simulink library "speedgoatlib_IO682_3210"  (R2024b)
settings: Solver=FixedStepAuto  StartTime=0.0  StopTime=10.0  RelTol=1e-3  EnableMultiTasking=on
undefined symbols (not defined in the file): sg_io682_receive_decode_m_v2
libraries: speedgoatlib_obsolete x1
settings Model: Creator=cschafft  LastModifiedBy=speedgoat\jenkins
settings SolverCC: ConcurrentTasks=on  AlgebraicLoopSolver=TrustRegion  AutoInsertRateTranBlk=on  InsertRTBMode=Never (minimum delay)
settings DataIOCC: LimitDataPoints=on  SaveFormat=StructureWithTime  ReturnWorkspaceOutputs=off
settings OptimizationCC: BlockReduction=off  OptimizeBlockIOStorage=off  BufferReuse=off  ReuseModelBlockBuffer=off  GlobalBufferReuse=off  ExpressionFolding=off  LocalBlockOutputs=off  OptimizeDataStoreBuffers=off  BusAssignmentInplaceUpdate=off
settings DebuggingCC: UnconnectedInputMsg=warning  UnconnectedOutputMsg=warning  UnconnectedLineMsg=warning  AllowSymbolicDim=off  SFUnexpectedBacktrackingDiag=warning  SFNoUnconditionalDefaultTransitionDiag=warning  SFExecutionAtInitializationDiag=none  ArithmeticOperatorsInVariantConditions=warning
settings HardwareCC: ProdBitPerPointer=32  ProdBitPerSizeT=32  ProdBitPerPtrDiffT=32  ProdLargestAtomicFloat=None  ProdWordSize=32  ProdLongLongMode=on  ProdHWDeviceType=Generic->32-bit x86 compatible
settings ModelReferenceCC: EnableRefExpFcnMdlSchedulingChecks=on  PropagateSignalLabelsOutOfModel=off
settings SFSimCC: SimUseLocalCustomCode=off  CustomCodeUndefinedFunction=UseInterfaceOnly
settings RTWCC: Description=Simulink Real-Time  SystemTargetFile=slrt.tlc  TemplateMakefile=slrt_default_tmf  RTWUseLocalCustomCode=off  RTWCompilerOptimization=on  GPUComputeCapability=3.5  DLArmComputeVersion=19.05
settings CodeAppCC: StateflowObjectComments=on
settings SimulinkRealTimeCC: SubcomponentCodeInterfacePackaging=Reusable function  SupportVariableSizeSignals=on  InstructionSetFMA=off  OptimizeReductions=off  LogToMDFFile=off  RL32LogTETModifier=off
settings ConfigComp: CovMetricSettings=dw  CovSaveCumulativeToWorkspaceVar=on  CovSaveSingleToWorkspaceVar=on  CovExternalEMLEnable=off  CovBoundaryAbsTol=1.0e-5

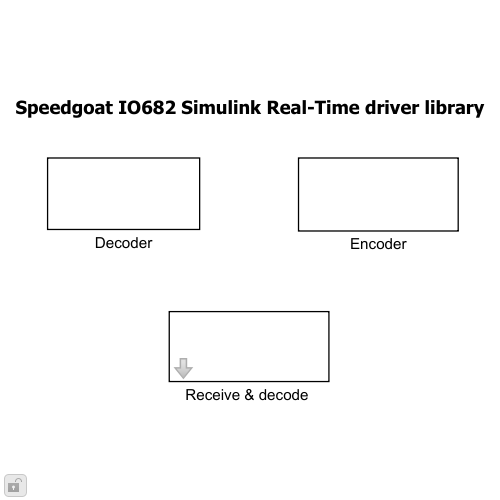
[thumbnail: Simulink's stored preview of the top-level diagram]
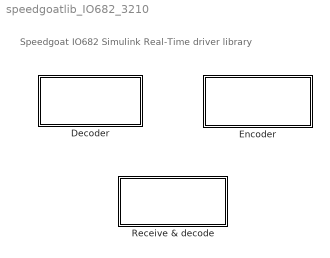
== system speedgoatlib_IO682_3210 ==
  note: Speedgoat IO682 Simulink Real-Time driver library
  Decoder : Subsystem
  Encoder : Subsystem
  "Receive & decode " : Subsystem  InitFcn=sg_io682_receive_decode_m_v2.runInitFcn();  mask(receive_decode_IO682){parChannel=1, parImportedIcdFile=, parSampleTime=-1, parSelectedLabels=[]}
      mask prompts: parChannel "Channel"; parImportedIcdFile "Available Messages (*.csv)"; parSampleTime "Sample Time [s]"
      mask help:
      | Receive and decode data from ARINC 429.
      | Use the "Select Messages to Decode" button to select the messages to decode, the block will automatically configure itself based on label name. The message description is given by the ICD file defined in "Available Messages".
      mask init:
      | sg_io682_receive_decode_m_v2.runMaskInitialization();
      settings: CopyFcn=sg_io682_receive_decode_m_v2.runCopyFcn();
      mask TypeOptions parChannel: Receive v2 /parChannel
      mask TypeOptions parSampleTime: Receive v2 /parSampleTime
      mask DialogControl parImportIcdFile Prompt: Browse
      mask DialogControl parImportIcdFile Callback: sg_io682_receive_decode_m_v2.runImportIcdFileCb();
      mask DialogControl parSelectLabels Prompt: Select Messages to Decode
      mask DialogControl parSelectLabels Callback: sg_io682_receive_decode_m_v2.runSelectLabelsCb();

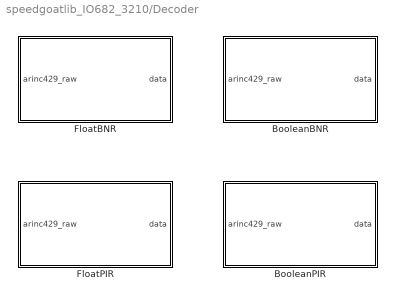
== system speedgoatlib_IO682_3210/Decoder ==
  BooleanBNR : Subsystem  mask(Boolean BNR Decoder){label=0, float_resolution=0, signal_lsb=0, signal_msb=0}
      mask prompts: float_resolution "Float Resolution"; signal_lsb "Signal LSB"; signal_msb "Signal MSB"
      mask help: Decode an ARINC message in BNR format of boolean data type.
  BooleanPIR : Subsystem  mask(Boolean PIR Decoder){label=0, float_resolution=0, signal_lsb=0, signal_msb=0}
      mask prompts: float_resolution "Float Resolution"; signal_lsb "Signal LSB"; signal_msb "Signal MSB"
      mask help: Decode an ARINC message of boolean data type when encoded as "Parameter In Demand" (PIR) using IEEE encoding.
  FloatBNR : Subsystem  mask(Float BNR Decoder){label=0, float_resolution=0, signal_lsb=0, signal_msb=0}
      mask prompts: float_resolution "Float Resolution"; signal_lsb "Signal LSB"; signal_msb "Signal MSB"
      mask help: Decode an ARINC message in BNR format of float data type.
  FloatPIR : Subsystem  mask(Float PIR Decoder){label=0, float_resolution=0, signal_lsb=0, signal_msb=0}
      mask prompts: float_resolution "Float Resolution"; signal_lsb "Signal LSB"; signal_msb "Signal MSB"
      mask help: Decode an ARINC message of float data type when encoded as "Parameter In Demand" (PIR) using IEEE encoding.

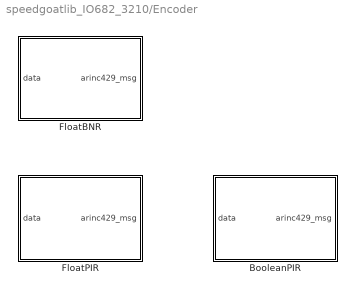
== system speedgoatlib_IO682_3210/Encoder ==
  BooleanPIR : Subsystem  mask(Boolean PIR Encoder){label=0, SSM=0, SDI=0}
      mask help: Encode an ARINC message from a boolean data as a "Parameter In Demand" (PIR) using the IEEE encoding.
  FloatBNR : Subsystem  mask(Float BNR Encoder){label=0, SSM=0, SDI=0, float_resolution=0, signal_lsb=0, signal_msb=0}
      mask prompts: float_resolution "Float Resolution"; signal_lsb "Signal LSB"; signal_msb "Signal MSB"
      mask help: Encode an ARINC message from a float data using the BNR encoding.
  FloatPIR : Subsystem  mask(Float PIR Encoder){label=0}
      mask help: Encode an ARINC message from a float data as a "Parameter In Demand" (PIR) using the IEEE encoding.

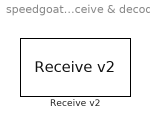
== system speedgoatlib_IO682_3210/Receive & decode  ==
  "Receive v2 " : speedgoatlib_obsolete/IO682/Receive v2   parModuleId=1  parChannel=1  parMaxWords=50  parMinWords=1  parSampleTime=parSampleTime

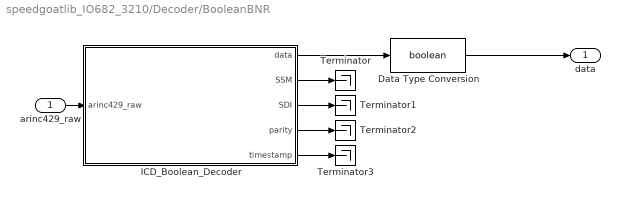
== system speedgoatlib_IO682_3210/Decoder/BooleanBNR ==
  arinc429_raw : Inport
  Data Type Conversion : DataTypeConversion  OutDataTypeStr=boolean  SaturateOnIntegerOverflow=off  RndMeth=Floor
  ICD_Boolean_Decoder : MATLAB Function  TreatAsAtomicUnit=on  VariantControl=mode==99
  Terminator{,1..3} (4 alike) : Terminator
  data : Outport  VectorParamsAs1DForOutWhenUnconnected=off
  wires:
  arinc429_raw/1 -> ICD_Boolean_Decoder/1(arinc429_raw)
  ICD_Boolean_Decoder/1(data) -> Data Type Conversion/1
  ICD_Boolean_Decoder/2(SSM) -> Terminator/1
  ICD_Boolean_Decoder/3(SDI) -> Terminator1/1
  ICD_Boolean_Decoder/4(parity) -> Terminator2/1
  ICD_Boolean_Decoder/5(timestamp) -> Terminator3/1
  Data Type Conversion/1 -> data/1

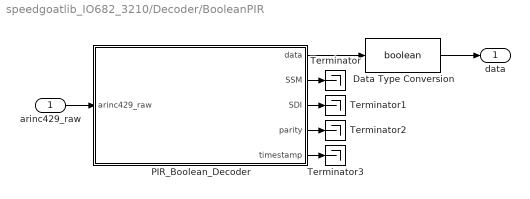
== system speedgoatlib_IO682_3210/Decoder/BooleanPIR ==
  arinc429_raw : Inport
  Data Type Conversion : DataTypeConversion  OutDataTypeStr=boolean  SaturateOnIntegerOverflow=off  RndMeth=Floor
  PIR_Boolean_Decoder : MATLAB Function  TreatAsAtomicUnit=on
  Terminator{,1..3} (4 alike) : Terminator
  data : Outport  VectorParamsAs1DForOutWhenUnconnected=off
  wires:
  arinc429_raw/1 -> PIR_Boolean_Decoder/1(arinc429_raw)
  PIR_Boolean_Decoder/2(SSM) -> Terminator/1
  PIR_Boolean_Decoder/1(data) -> Data Type Conversion/1
  PIR_Boolean_Decoder/3(SDI) -> Terminator1/1
  PIR_Boolean_Decoder/4(parity) -> Terminator2/1
  PIR_Boolean_Decoder/5(timestamp) -> Terminator3/1
  Data Type Conversion/1 -> data/1

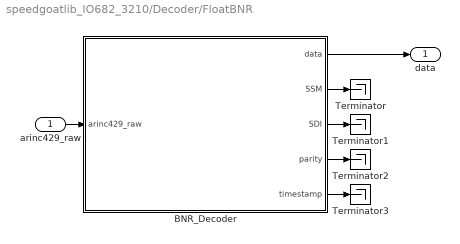
== system speedgoatlib_IO682_3210/Decoder/FloatBNR ==
  arinc429_raw : Inport
  BNR_Decoder : MATLAB Function  TreatAsAtomicUnit=on  VariantControl=mode==99
  Terminator{,1..3} (4 alike) : Terminator
  data : Outport  VectorParamsAs1DForOutWhenUnconnected=off
  wires:
  BNR_Decoder/5(timestamp) -> Terminator3/1
  BNR_Decoder/1(data) -> data/1
  BNR_Decoder/2(SSM) -> Terminator/1
  BNR_Decoder/3(SDI) -> Terminator1/1
  arinc429_raw/1 -> BNR_Decoder/1(arinc429_raw)
  BNR_Decoder/4(parity) -> Terminator2/1

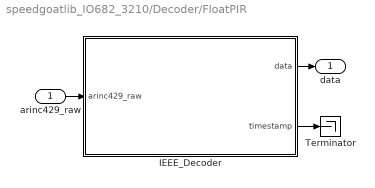
== system speedgoatlib_IO682_3210/Decoder/FloatPIR ==
  arinc429_raw : Inport
  IEEE_Decoder : MATLAB Function  TreatAsAtomicUnit=on
  Terminator : Terminator
  data : Outport  VectorParamsAs1DForOutWhenUnconnected=off
  wires:
  IEEE_Decoder/1(data) -> data/1
  arinc429_raw/1 -> IEEE_Decoder/1(arinc429_raw)
  IEEE_Decoder/2(timestamp) -> Terminator/1

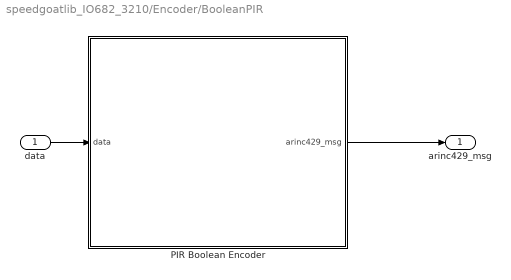
== system speedgoatlib_IO682_3210/Encoder/BooleanPIR ==
  data : Inport
  PIR Boolean Encoder : MATLAB Function  TreatAsAtomicUnit=on
  arinc429_msg : Outport  VectorParamsAs1DForOutWhenUnconnected=off
  wires:
  PIR Boolean Encoder/1(arinc429_msg) -> arinc429_msg/1
  data/1 -> PIR Boolean Encoder/1(data)

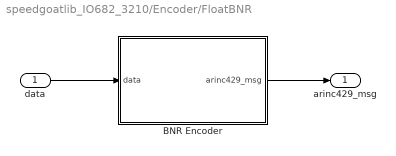
== system speedgoatlib_IO682_3210/Encoder/FloatBNR ==
  data : Inport
  BNR Encoder : MATLAB Function  TreatAsAtomicUnit=on
  arinc429_msg : Outport  VectorParamsAs1DForOutWhenUnconnected=off
  wires:
  data/1 -> BNR Encoder/1(data)
  BNR Encoder/1(arinc429_msg) -> arinc429_msg/1

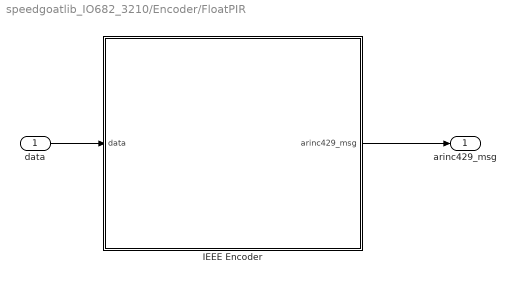
== system speedgoatlib_IO682_3210/Encoder/FloatPIR ==
  data : Inport
  IEEE Encoder : MATLAB Function  TreatAsAtomicUnit=on
  arinc429_msg : Outport  VectorParamsAs1DForOutWhenUnconnected=off
  wires:
  data/1 -> IEEE Encoder/1(data)
  IEEE Encoder/1(arinc429_msg) -> arinc429_msg/1

== matlab function speedgoatlib_IO682_3210/Decoder/FloatBNR/BNR_Decoder ==
  data: arinc429_raw input double; label parameter int32; data output size=[1, 1]; float_resolution parameter double size=[1, 1]; signal_lsb parameter int32 size=[1, 1]; signal_msb parameter int32 size=[1, 1]; SSM output; SDI output; parity output; timestamp output
% Function description: this function takes a vector of ARINC429 as inputs
% and decodes its content.
%
% 
%
%
function [data,SSM,SDI,parity,timestamp] = fcn(arinc429_raw, label, float_resolution, signal_lsb, signal_msb)
%#codegen

persistent data_buf;
persistent SDI_buf;
persistent SSM_buf;
persistent timestamp_buf;

if isempty(data_buf)
    data_buf = double(0.0);
end

if isempty(SDI_buf)
    SDI_buf = double(0.0);
end

if isempty(SSM_buf)
    SSM_buf = double(0.0);
end

if isempty(timestamp_buf)
    timestamp_buf = double(0.0);
end
    

% We process all the inputs messages and if the labels matches, then the
% buffered variables (_buf) are updated.

% When no label match, we keep the values of the previous execution
for i = 1:length(arinc429_raw)

    arinc429_raw_64 = typecast(arinc429_raw(i), 'uint64');
    arinc429_raw_32_low = uint32(bitand(arinc429_raw_64, 2^32-1));
    arinc429_raw_32_high = uint32(bitand(bitshift(arinc429_raw_64, -32), 2^32-1));

    label_field = int32(bitand(arinc429_raw_32_low, uint32(255)));

    if label_field == label

        % Index the bits position from offset 0.
        signal_lsb = signal_lsb - 1;
        signal_msb = signal_msb - 1;
        signal_range = signal_msb - signal_lsb + 1;

        % Get the sign (bit 29)
        sign = bitand(bitshift(arinc429_raw_32_low, -signal_msb -1), 1);

        % Get the data field
        data_bnr_mask = uint32(2^(signal_range) - 1);
        data_bnr = uint32(arinc429_raw_32_low);
        data_bnr = bitand(bitshift(data_bnr, -signal_lsb), data_bnr_mask);        

        % If needed, pad the sign bit (we work on 32-bits)
        if sign > 0
            % fill all the bits between sign and MSB with logic 1
            padding_bits = uint32(bitshift(uint32(2^(32 - signal_range) - 1), signal_range));
            data_bnr_signed = typecast(bitor(data_bnr, padding_bits), 'int32');
        else
            data_bnr_signed = typecast(data_bnr, 'int32');    
        end
        
        % Get the SSM field
        SSM_buf = double(bitand(bitshift(arinc429_raw_32_low, -29), 3));
        
        % Get the SDI field
        SDI_buf = double(bitand(bitshift(arinc429_raw_32_low, -8), 3));

        % Update the data only when labels match
        data_buf = double(float_resolution * double(data_bnr_signed));
        timestamp_buf = double(arinc429_raw_32_high);


    end

end


% Update the output using the buffered values.
data = data_buf;
SSM = SSM_buf;
SDI = SDI_buf;
parity = -1.0;
timestamp = timestamp_buf;

== matlab function speedgoatlib_IO682_3210/Decoder/FloatPIR/IEEE_Decoder ==
  data: data output double size=[1, 1]; arinc429_raw input double; timestamp output; label parameter
function [data, timestamp]  = fcn(arinc429_raw, label)
%#codegen

% Function description: this function takes a vector of ARINC429 as inputs
% and decodes its content.

persistent data_buf;
persistent timestamp_buf;

if isempty(data_buf)
    data_buf = double(0.0);
end
    

if isempty(timestamp_buf)
    timestamp_buf = double(0.0);
end
    

% We process all the inputs messages and if the labels matches, then the
% buffered variables (_buf) are updated.

% When no label match, we keep the values of the previous execution
for i = 1:length(arinc429_raw)

    arinc429_raw_64 = typecast(arinc429_raw(i), 'uint64');
    arinc429_raw_32_low = uint32(bitand(arinc429_raw_64, 2^32-1));
    arinc429_raw_32_high = uint32(bitand(bitshift(arinc429_raw_64, -32), 2^32-1));

    label_field = int32(bitand(arinc429_raw_32_low, uint32(255)));

    if label_field == label

        % Get the sign (bit 31)
        sign = bitand(bitshift(arinc429_raw_32_low, -30), 1);

        % Get the exponent and the mantissa
        exponent =  int32(bitand(bitshift(arinc429_raw_32_low, -22), 255)) - 127;        
        mantissa_bnr = uint32(bitand(bitshift(arinc429_raw_32_low, -8), 2^14-1));
        mantissa = 0.0;
        for j = 1:14
            if bitand(mantissa_bnr, 8192)
                mantissa = mantissa + 2^(-j);
            end
            mantissa_bnr = bitshift(mantissa_bnr, 1);
        end
        mantissa = mantissa + 1;
        
        % Update the data only when labels match
        data_buf = double((-1.0)^double(sign) * 2^(double(exponent)) * double(mantissa));
        timestamp_buf = double(arinc429_raw_32_high);


    end

end


% Update the output using the buffered values.
data = data_buf;
timestamp = timestamp_buf;

== matlab function speedgoatlib_IO682_3210/Decoder/BooleanBNR/ICD_Boolean_Decoder ==
  data: arinc429_raw input double; label parameter int32; data output size=[1, 1]; signal_lsb parameter int32 size=[1, 1]; signal_msb parameter int32 size=[1, 1]; SSM output; SDI output; parity output; timestamp output
% Function description: this function takes a vector of ARINC429 as inputs
% and decodes its content.
%
% 
%
%
function [data,SSM,SDI,parity,timestamp] = fcn(arinc429_raw, label, signal_lsb, signal_msb)
%#codegen

persistent data_buf;
persistent SDI_buf;
persistent SSM_buf;
persistent timestamp_buf;

if isempty(data_buf)
    data_buf = double(0.0);
end

if isempty(SDI_buf)
    SDI_buf = double(0.0);
end

if isempty(SSM_buf)
    SSM_buf = double(0.0);
end

if isempty(timestamp_buf)
    timestamp_buf = double(0.0);
end
    

% We process all the inputs messages and if the labels matches, then the
% buffered variables (_buf) are updated.

% When no label match, we keep the values of the previous execution
for i = 1:length(arinc429_raw)

    arinc429_raw_64 = typecast(arinc429_raw(i), 'uint64');
    arinc429_raw_32_low = uint32(bitand(arinc429_raw_64, 2^32-1));
    arinc429_raw_32_high = uint32(bitand(bitshift(arinc429_raw_64, -32), 2^32-1));

    label_field = int32(bitand(arinc429_raw_32_low, uint32(255)));

    if label_field == label

        % Index the bits position from offset 0.
        signal_lsb = signal_lsb - 1;
        signal_msb = signal_msb - 1;
        signal_range = signal_msb - signal_lsb + 1;

        % Get the sign (bit 29)
        sign = bitand(bitshift(arinc429_raw_32_low, -signal_msb -1), 1);

        % Get the data field
        data_bnr_mask = uint32(2^(signal_range) - 1);
        data_bnr = uint32(arinc429_raw_32_low);
        data_bnr = bitand(bitshift(data_bnr, -signal_lsb), data_bnr_mask);        

        % If needed, pad the sign bit (we work on 32-bits)
        if sign > 0
            % fill all the bits between sign and MSB with logic 1
            padding_bits = uint32(bitshift(uint32(2^(32 - signal_range) - 1), signal_range));
            data_bnr_signed = typecast(bitor(data_bnr, padding_bits), 'int32');
        else
            data_bnr_signed = typecast(data_bnr, 'int32');    
        end
        
        % Get the SSM field
        SSM_buf = double(bitand(bitshift(arinc429_raw_32_low, -29), 3));
        
        % Get the SDI field
        SDI_buf = double(bitand(bitshift(arinc429_raw_32_low, -8), 3));

        % Update the data only when labels match       
        data_buf = double(double(data_bnr_signed));
        timestamp_buf = double(arinc429_raw_32_high);


    end

end

% Update the output using the buffered values.
data = data_buf;
SSM = SSM_buf;
SDI = SDI_buf;
parity = -1.0;
timestamp = timestamp_buf;

== matlab function speedgoatlib_IO682_3210/Encoder/BooleanPIR/PIR Boolean Encoder ==
  data: data input double size=[1, 1]; arinc429_msg output double size=[1, 1]; SSM parameter uint32 size=[1, 1]; SDI parameter uint32 size=[1, 1]; label parameter uint32 size=[1, 1]
function arinc429_msg = fcn(data, SSM, SDI, label)
%#codegen
% Scale the data using the float resolution parameter.

if data > 0.5
    data_32 = uint32(2^21);
else
    data_32 = uint32(0);
end   

label = bitand(label, bin2dec('00000000000000000000000011111111'));
SDI = bitand(SDI, bin2dec('00000000000000000000000000000011'));
SSM = bitand(SSM, bin2dec('00000000000000000000000000000011'));

arinc429_32 = uint32(bitor(bitshift(SSM, 29), bitor(bitshift(SDI, 8), bitor(data_32, label))));
arinc429_64 = uint64(arinc429_32);
arinc429_msg = typecast(arinc429_64, 'double');

== matlab function speedgoatlib_IO682_3210/Encoder/FloatBNR/BNR Encoder ==
  data: data input double size=[1, 1]; arinc429_msg output double size=[1, 1]; SSM parameter uint32 size=[1, 1]; SDI parameter uint32 size=[1, 1]; label parameter uint32 size=[1, 1]; float_resolution parameter; signal_lsb parameter; signal_msb parameter
function arinc429_msg = bnr_encoder(data, SSM, SDI, label, float_resolution, signal_lsb, signal_msb)
%#codegen
% Scale the data using the float resolution parameter.
signal_lsb = signal_lsb - 1;
data_32 = typecast(int32(data / float_resolution), 'uint32');
data_32 = bitshift(data_32, signal_lsb);    

label = bitand(label, bin2dec('00000000000000000000000011111111'));
SDI = bitand(SDI, bin2dec('00000000000000000000000000000011'));
SSM = bitand(SSM, bin2dec('00000000000000000000000000000011'));

arinc429_32 = uint32(bitor(bitshift(SSM, 29), bitor(bitshift(SDI, 8), bitor(data_32, label))));
sign = bitand(bitshift(arinc429_32, -28), 1)
arinc429_64 = uint64(arinc429_32);
arinc429_msg = typecast(arinc429_64, 'double');

== matlab function speedgoatlib_IO682_3210/Decoder/BooleanPIR/PIR_Boolean_Decoder ==
  data: arinc429_raw input double; label parameter uint32; data output size=[1, 1]; SSM output double size=[1, 1]; SDI output double size=[1, 1]; parity output double size=[1, 1]; timestamp output
% Function description: this function takes a vector of ARINC429 as inputs
% and decodes its content.
%
% 
%
%
function [data, SSM, SDI, parity, timestamp] = fcn(arinc429_raw, label)
%#codegen
bool_pos = 22 - 1;
persistent data_buf;
persistent SDI_buf;
persistent SSM_buf;
persistent timestamp_buf;

if isempty(data_buf)
    data_buf = false;
end

if isempty(SDI_buf)
    SDI_buf = double(0.0);
end

if isempty(SSM_buf)
    SSM_buf = double(0.0);
end

if isempty(timestamp_buf)
    timestamp_buf = double(0.0);
end
    

% We process all the inputs messages and if the labels matches, then the
% buffered variables (_buf) are updated.

% When no label match, we keep the values of the previous execution
for i = 1:length(arinc429_raw)

    arinc429_raw_64 = typecast(arinc429_raw(i), 'uint64');
    arinc429_raw_32_low = uint32(bitand(arinc429_raw_64, 2^32-1));
    arinc429_raw_32_high = uint32(bitand(bitshift(arinc429_raw_64, -32), 2^32-1));

    label_field = int32(bitand(arinc429_raw_32_low, uint32(255)));

    if label_field == label       
     
        % Update the data only when labels match
        if bitand(bitshift(arinc429_raw_32_low, -bool_pos), 1) > 0        
            data_buf = true;
        else
            data_buf = false;
        end
        
        timestamp_buf = double(arinc429_raw_32_high);

    end

end


% Update the output using the buffered values.
data = double(data_buf);
SSM = SSM_buf;
SDI = SDI_buf;
parity = -1.0;
timestamp = timestamp_buf;

== matlab function speedgoatlib_IO682_3210/Encoder/FloatPIR/IEEE Encoder ==
  data: data input double size=[1, 1]; arinc429_msg output double size=[1, 1]; label parameter uint32 size=[1, 1]
function arinc429_msg  = fcn(data, label)
%#codegen

 mantissa_bnr = uint32(0);

    % Determination du signe
    if data < 0
        sign = 1;
    else
        sign = 0;
    end
    
    % Aucun codage supplémentaire pour les nombres négatifs (le signe étant déjà extrait)
    data = abs(data);
    
    % calcul de l'exposant:
    % le but est de représenter la valeur par: m * 2(exposant) et où m est
    % compris entre 1 et 2 (ou en d'autres mots 1+fraction)
    
    % On divise donc la valeur (data) par tous les exposants disponibles
    % pour trouver une base (1 + fraction) entre 1 et 2.    
    
    exponent = double(ceil(log(data / 2) / log(2) + 127)); % Ajout du bias pour un coder une éventuelle puissance négative.
    mantissa = data / 2^(exponent - 127) - 1;
    
    % la mantisse doit être représentée par une somme (2^-1 + 2^-2 ... + 2^-14)
    mantissa_work = mantissa;
    for i = 1:14
        mantissa_work = mantissa_work * 2;        
        if mantissa_work >= 1
            mantissa_work = mantissa_work - 1;
            mantissa_bnr = bitshift(mantissa_bnr, 1) + 1;
        else
            mantissa_bnr = bitshift(mantissa_bnr, 1);
        end
        
    end
        
    data_256 = uint32(bitor(bitor(bitshift(mantissa_bnr, 8), bitor(bitshift(sign, 30), bitshift(uint32(exponent), 22))), uint32(label)));
    
    arinc429_64 = uint64(data_256);
    arinc429_msg = typecast(arinc429_64, 'double');
